simulink model "Lead_Compensator_DC_Motor_Model"  (R2021a)
settings: Solver=VariableStepAuto  StartTime=0.0  StopTime=30  RelTol=1e-3
values from neighbouring files (symbols this model uses):
  b = 0.0408    [Lead_Compensator_DC_Motor.m]
  gain = alpha    [Lead_Compensator_DC_Motor.m]
  J = 3    [Lead_Compensator_DC_Motor.m]
  Kb = 0.929    [Lead_Compensator_DC_Motor.m]
  Kt = 0.929    [Lead_Compensator_DC_Motor.m]
  L = 0.2    [Lead_Compensator_DC_Motor.m]
  R = 0.5    [Lead_Compensator_DC_Motor.m]
settings Model: Creator=Electrical Dept  LastModifiedBy=mofid
settings SolverCC: AlgebraicLoopSolver=TrustRegion
settings SFSimCC: CustomCodeUndefinedFunction=UseInterfaceOnly
settings RTWCC: DLArmComputeVersion=20.02.1

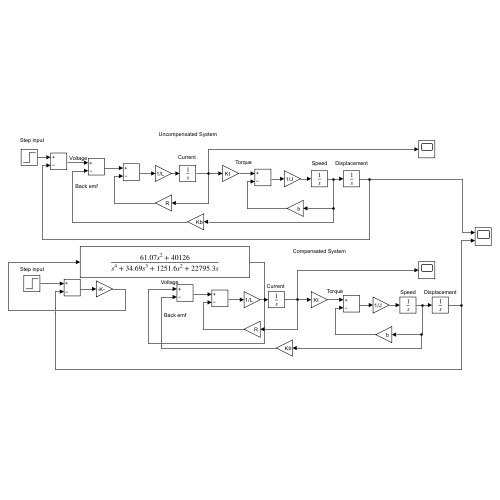
[thumbnail: Simulink's stored preview of the top-level diagram]
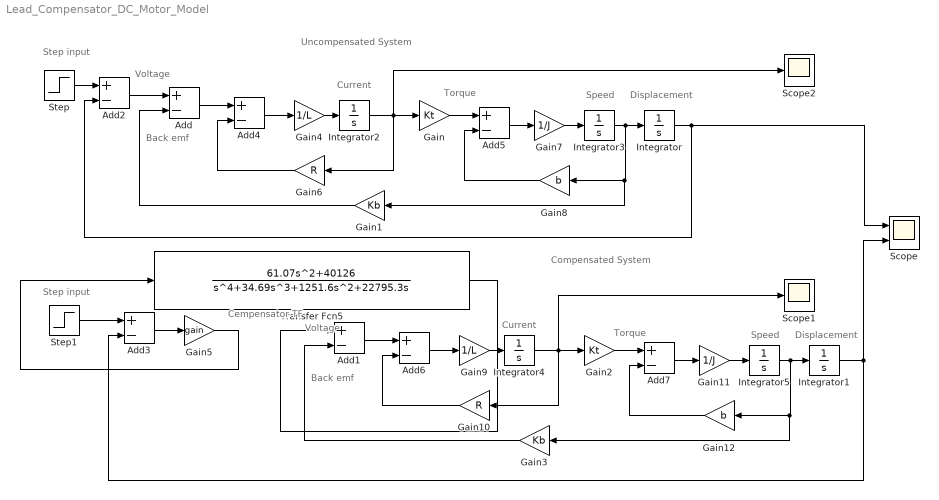
== system Lead_Compensator_DC_Motor_Model ==
  note: Voltage
  note: Back emf
  note: Torque
  note: Step input
  note: Cempensator TF
  note: Current
  note: Displacement
  note: Speed
  note: Compensated System
  note: Uncompensated System
  note: Current
  note: Speed
  note: Displacement
  note: Step input
  note: Torque
  note: Back emf
  note: Voltage
  Add{,1..7} (8 alike) : Sum  Inputs=+-
  Gain : Gain  Gain=Kt
  Gain1 : Gain  Gain=Kb
  Gain10 : Gain  Gain=R
  Gain11 : Gain  Gain=1/J
  Gain12 : Gain  Gain=b
  Gain2 : Gain  Gain=Kt
  Gain3 : Gain  Gain=Kb
  Gain4 : Gain  Gain=1/L
  Gain5 : Gain  Gain=gain
  Gain6 : Gain  Gain=R
  Gain7 : Gain  Gain=1/J
  Gain8 : Gain  Gain=b
  Gain9 : Gain  Gain=1/L
  Integrator{,1..5} (6 alike) : Integrator
  Scope : Scope  NumInputPorts=2
  Scope1 : Scope
  Scope2 : Scope
  Step : Step  Time=0  SampleTime=0
  Step1 : Step  Time=0  SampleTime=0
  Transfer Fcn5 : TransferFcn  Numerator=[61.07 0 40126]  Denominator=[1 34.69 1251.6 22795.3 0]
  wires:
  Add/1 -> Add4/1
  Integrator2/1 -> Gain/1, Gain6/1, Scope2/1
  Gain1/1 -> Add/2
  Integrator/1 -> Add2/2, Scope/1
  Step/1 -> Add2/1
  Add2/1 -> Add/1
  Step1/1 -> Add3/1
  Gain5/1 -> Transfer Fcn5/1
  Add3/1 -> Gain5/1
  Add4/1 -> Gain4/1
  Gain6/1 -> Add4/2
  Gain4/1 -> Integrator2/1
  Gain/1 -> Add5/1
  Gain8/1 -> Add5/2
  Add5/1 -> Gain7/1
  Gain7/1 -> Integrator3/1
  Integrator3/1 -> Gain1/1, Gain8/1, Integrator/1
  Add7/1 -> Gain11/1
  Gain12/1 -> Add7/2
  Gain10/1 -> Add6/2
  Add6/1 -> Gain9/1
  Add1/1 -> Add6/1
  Gain3/1 -> Add1/2
  Gain2/1 -> Add7/1
  Integrator5/1 -> Gain3/1, Gain12/1, Integrator1/1
  Gain9/1 -> Integrator4/1
  Transfer Fcn5/1 -> Add1/1
  Integrator4/1 -> Gain2/1, Gain10/1, Scope1/1
  Gain11/1 -> Integrator5/1
  Integrator1/1 -> Scope/2, Add3/2
